simulink model "test_sys_characteristics"  (R2019a)
settings: Solver=FixedStepAuto  StartTime=0.0  StopTime=Tend  FixedStep=ts  RelTol=1e-3
values from neighbouring files (symbols this model uses):
  den = [1 1]    [test_Tfm.m]    (also in zhujiaqi_1911056.m)
  num = [1]    [test_Tfm.m]    (also in zhujiaqi_1911056.m)
  Tend = 40    [mian1.m]    (also in test_Tfm.m)
  w1 = fmax*2*pi    (= 0.948760981384)    [mian1.m]    (also in test_Tfm.m)
libraries: simulink x1
settings Model: Creator=lzr96  LastModifiedBy=lzr96

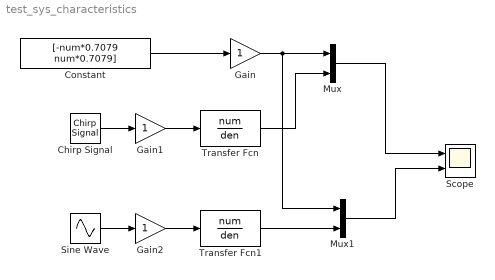
== system test_sys_characteristics ==
  Chirp Signal : simulink/Sources/Chirp Signal  f1=Fstart  T=Tend  f2=Fend
  Constant : Constant  Value=[-num*0.7079 num*0.7079]
  Gain : Gain
  Gain1 : Gain
  Gain2 : Gain
  Mux : Mux  Inputs=2
  Mux1 : Mux  Inputs=2
  Scope : Scope  NumInputPorts=2
  Sine Wave : Sin  Frequency=w1  SampleTime=0
  Transfer Fcn : TransferFcn  Numerator=num  Denominator=den
  Transfer Fcn1 : TransferFcn  Numerator=num  Denominator=den
  wires:
  Chirp Signal/1 -> Gain1/1
  Sine Wave/1 -> Gain2/1
  Constant/1 -> Gain/1
  Gain/1 -> Mux1/1, Mux/1
  Transfer Fcn/1 -> Mux/2
  Transfer Fcn1/1 -> Mux1/2
  Mux/1 -> Scope/1
  Mux1/1 -> Scope/2
  Gain1/1 -> Transfer Fcn/1
  Gain2/1 -> Transfer Fcn1/1
